simulink library "util_extra_lib"  (R2014b)
settings: Solver=ode45  StartTime=0.0  StopTime=10.0  RelTol=1e-3
values from neighbouring files (symbols this model uses):
  dt = 0.1    [quat_prop_test.m]
undefined symbols (not defined in the file or in its folder): duty_dt, min_dt, Newton, Raphson
undefined symbols (not defined in the file): asq_sequencer_rate, csc_gdn_dt, csu_rbd_orientation_prep_pitch_transfer_den, csu_rbd_orientation_prep_pitch_transfer_num
libraries: simulink x9, util_extra_lib x5, util_common_lib x1
settings Model: Creator=ianmga  LastModifiedBy=mstewart

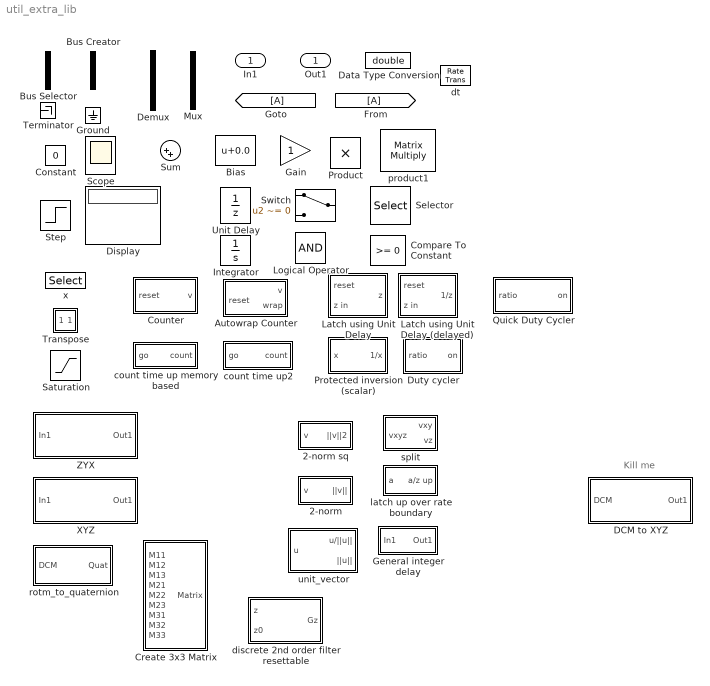
== system util_extra_lib ==
  note: Kill me
  In1 : Inport
  2-norm : Subsystem
  2-norm sq : Subsystem
  Autowrap Counter : Subsystem  mask{dt=dt, v0=int32( 0 ), dv=int32( 1 ), vlimit=int32( duty_dt / dt )}
      mask prompts: dt "Sample rate [s]"; v0 "Initial value"; dv "Increment"; vlimit "Wrap limit"
  Bias : Bias  Bias=0.0
  Bus Creator : BusCreator  Inputs=2
  Bus Selector : BusSelector  OutputSignals=signal1,signal2
  Compare To Constant : simulink/Logic and Bit Operations/Compare To Constant  relop=>=  const=0  OutDataTypeStr=uint8
  Constant : Constant  Value=0
  Counter : Subsystem  mask{dt=csc_gdn_dt, v0=0, dv=csc_gdn_dt}
      mask prompts: dt "Sample rate [s]"; v0 "Initial value"; dv "Increment"
  Create 3x3 Matrix : Subsystem  mask(Create 3x3 Matrix){}
      mask help:
      | Create a 3-by-3 matrix from nine input values. Each input corresponds to an element of the matrix.
      |
      | For example, the input labeled A21 is the entry in the second row and first column of the matrix.
      mask Help: eval('asbhelp(''create_threebythree_matrix'')');
      mask Display:
      | port_label('input',1,'A_{11}','texmode','on');
      | port_label('input',2,'A_{12}','texmode','on');
      | port_label('input',3,'A_{13}','texmode','on');
      | port_label('input',4,'A_{21}','texmode','on');
      | port_label('input',5,'A_{22}','texmode','on');
      | port_label('input',6,'A_{23}','texmode','on');
      | port_label('input',7,'A_{31}','texmode','on');
      | port_label('input',8,'A_{32}','texmode','on');
      | port_label('input',9,'A_{33}','texmode','on');
      | port_label('output',1,'A','texmode','on');
  DCM to XYZ : Subsystem  mask(DCM2Ang){}
      mask help:
      | Determine rotation vector from the 3-by-3 direction cosine matrix (DCM).
      |
      | The 'Default' limitations for the 'ZYX', 'ZXY', 'YXZ', 'YZX', 'XYZ', and 'XZY' implementations generate an R2 angle that lies between +/- 90 degrees, and R1 and R3 angles that lie between +/- 180 degrees.
      |
      | The 'Default' limitations for the 'ZYZ', 'ZXZ', 'YXY', 'YZY', 'XYX', and 'XZX' implementations generate an R2 angle that lies between 0 and 180 degrees, and R1 and R3 angles that lie between +/- 180 degrees.
      |
      | The 'ZeroR3' limitations for the 'ZYX', 'ZXY', 'YXZ', 'YZX', 'XYZ', and 'XZY' implementations generate an R2 angle that lies between +/- 90 degrees, and R1 and R3 angles that lie between +/- 180 degrees. However, when R2 is +/- 90 degrees, R3 is set to 0 degrees.
      |
      | The 'ZeroR3' limitations for the 'ZYZ', 'ZXZ', 'YXY', 'YZY', 'XYX', and 'XZX' implementations generate an R2 angle that lies between 0 and 180 degrees, and R1 and R3 angles that lie between +/- 180 degrees. However, when R2 is 0 or +/- 180 degrees, R3 is set to 0 degrees.
      mask Display:
      | port_label('input',1,'DCM^B_I','texmode','on')
      | port_label('output',1,'[R_X,R_Y,R_Z]','texmode','on')
  Data Type Conversion : DataTypeConversion  OutDataTypeStr=double
  Demux : Demux  Outputs=3
  Display : Display
  Duty cycler : Subsystem  mask{duty_dt=duty_dt, min_dt=min_dt, dt=dt}
      mask prompts: duty_dt "Duty cycle time [s]"; min_dt "Min duty cycle time [s]"; dt "Sample time [s]"
  Gain : Gain
  General integer delay : Subsystem  mask{delay_n=-1/.01, v0=0.0, dt=.01}
      mask prompts: delay_n "Delay samples"; v0 "Initial value"; dt "Sample time"
      mask Display:
      | port_label('input',1,'z');
      | port_label('output',1,'z^{-n}','texmode','on');
  Ground : Ground
  Integrator : Integrator
  Latch using Unit Delay : Subsystem  mask{z0=`, dt=dt}
      mask prompts: z0 "Initial value"; dt "Sample time"
  Latch using Unit Delay (delayed) : Subsystem  mask{z0=0, dt=dt}
      mask prompts: z0 "Initial value"; dt "Sample time"
  Logical Operator : Logic  AllPortsSameDT=off  OutDataTypeStr=boolean
  Mux : Mux  Inputs=3
  Product : Product  RndMeth=Zero
  Protected inversion (scalar) : Subsystem  mask{eps=1e-10}
  Quick Duty Cycler : Subsystem  mask{min_dt=0.1, dt=0.1}
      mask prompts: min_dt "Min duty cycle time [s]"; dt "Sample time [s]"
  Saturation : Saturate
  Scope : Scope  NumInputPorts=3
      settings: YMin=-5~-5~-5  YMax=5~5~5
  Selector : Selector  InputPortWidth=3  Indices=[1 3]
  Step : Step  SampleTime=0
  Sum : Sum  Inputs=|++
  Switch : Switch  Criteria=u2 ~= 0
  Terminator : Terminator
  Transpose : Subsystem  mask(Transpose){Hermitian=off, overflowFlag=off}
      mask prompts: overflowFlag "Saturate on integer overflow"
      mask help: Compute the matrix transpose. Vector input signals are treated as [Mx1] matrices. The output is always a matrix.
      mask init:
      | if(Hermitian==1)
      |     str = 'u^H';
      |     set_param([gcb '/Math Function'],'Operator','hermitian');
      |     if (overflowFlag==1)
      |         set_param([gcb '/Math Function'],'SaturateOnIntegerOverflow','on');
      |     else
      |         set_param([gcb '/Math Function'],'SaturateOnIntegerOverflow','off');
      |     end
      | else
      |     str = 'u^T';
      |     set_param([gcb '/Math Function'],'Operator','transpose');
      | end
      mask Help: eval('blocksethelp');
      mask Callback Hermitian:
      | if (strcmp(get_param(gcbh,'Hermitian'),'on'))
      | 	set_param(gcbh,'MaskVisibilities',{'on','on'});
      | else
      | 	set_param(gcbh,'MaskVisibilities',{'on','off'});
      | end
      mask Display: disp(str,'texmode','on')
  Unit Delay : UnitDelay  SampleTime=-1
  XYZ : Subsystem  mask(Ang2DCM){}
      mask help: Determine the 3-by-3 direction cosine matrix (DCM) from a given set of rotation angles.
      mask Display:
      | port_label('input',1,'[R_X,R_Y,R_Z]','texmode','on')
      | port_label('output',1,'DCM^B_I','texmode','on')
  ZYX : Subsystem  mask(Ang2DCM){}
      mask help: Determine the 3-by-3 direction cosine matrix (DCM) from a given set of rotation angles.
      mask Display:
      | port_label('input',1,'[R_Z,R_Y,R_X]','texmode','on')
      | port_label('output',1,'DCM^B_I','texmode','on')
  count time up memory based : Subsystem  mask{incr=int32( 1 ), v0=int32( 0 )}
      mask prompts: incr "Increment"; v0 "Initial value"
  count time up2 : Subsystem  mask{incr=asq_sequencer_rate, v0=0.0, dt=asq_sequencer_rate}
      mask prompts: incr "Increment"; v0 "Initial value"; dt "Sample time step"
  discrete 2nd order filter resettable : Subsystem  mask{num=csu_rbd_orientation_prep_pitch_transfer_num, den=csu_rbd_orientation_prep_pitch_transfer_den, dt=-1}
      mask prompts: num "Transfer fn numerator coefficients (bi)"; den "Transfer fn denominator coefficients (ai) (a1=1)"; dt "Sample rate (s)"
  dt : RateTransition  OutPortSampleTime=csc_gdn_dt
  latch up over rate boundary : Subsystem  mask{dt=.01}
      mask prompts: dt "Output sample time"
  product1 : Product  Multiplication=Matrix(*)
  rotm_to_quaternion : Subsystem  mask(DCM2Quaternion){}
      mask help: Determine the 4x1 quaternion orientation vector from a 3-by-3 direction cosine matrix (DCM). The input DCM transforms vectors from geodetic earth or north-east-down (NED) axes to body axes.
      mask Display:
      | port_label('output',1,'q^B_A','texmode','on')
      | port_label('input',1,'rotm^B_A','texmode','on')
  "split " : Subsystem
      mask Display:
      | port_label('input',1,'v_3','texmode','on')
      | port_label('output',1,'v_{xy}','texmode','on')
      | port_label('output',2,'v_z','texmode','on')
  unit_vector : Subsystem
      mask Display:
      | color('blue')
      | text(0.05,0.02,'NASA',...
      |  	'HorizontalAlignment','Left',...
      | 	'VerticalAlignment','bottom')
  x : Selector  InputPortWidth=3  Indices=[1]
  Out1 : Outport

== system util_extra_lib/2-norm ==
  v : Inport
  2-norm sq : util_extra_lib/2-norm sq
  Math Function : Math  Operator=sqrt  SaturateOnIntegerOverflow=on
  ||v|| : Outport
  wires:
  Math Function/1 -> ||v||/1
  v/1 -> 2-norm sq/1
  2-norm sq/1 -> Math Function/1

== system util_extra_lib/2-norm sq ==
  v : Inport
  Dot Product : DotProduct  InputSameDT=on  OutDataTypeStr=Inherit: Inherit via internal rule
  ||v||2 : Outport
  wires:
  Dot Product/1 -> ||v||2/1
  v/1 -> Dot Product/1, Dot Product/2

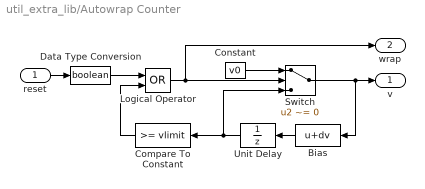
== system util_extra_lib/Autowrap Counter ==
  reset : Inport
  Bias : Bias  Bias=dv
  Compare To Constant : simulink/Logic and Bit Operations/Compare To Constant  relop=>=  const=vlimit  OutDataTypeStr=boolean
  Constant : Constant  Value=v0
  Data Type Conversion : DataTypeConversion  OutDataTypeStr=boolean
  Logical Operator : Logic  Operator=OR  AllPortsSameDT=off  OutDataTypeStr=boolean
  Switch : Switch  Criteria=u2 ~= 0  InputSameDT=on
  Unit Delay : UnitDelay  InitialCondition=vlimit  SampleTime=dt
  v : Outport
  wrap : Outport  Port=2
  wires:
  Data Type Conversion/1 -> Logical Operator/1
  Logical Operator/1 -> wrap/1, Switch/2
  reset/1 -> Data Type Conversion/1
  Compare To Constant/1 -> Logical Operator/2
  Constant/1 -> Switch/1
  Switch/1 -> Bias/1, v/1
  Bias/1 -> Unit Delay/1
  Unit Delay/1 -> Compare To Constant/1, Switch/3

== system util_extra_lib/Counter ==
  reset : Inport
  Bias : Bias  Bias=dv
  Constant : Constant  Value=v0  SampleTime=dt
  Switch : Switch  Criteria=u2 ~= 0  InputSameDT=on
  Unit Delay : UnitDelay  InitialCondition=v0  SampleTime=dt
  v : Outport
  wires:
  reset/1 -> Switch/2
  Unit Delay/1 -> Switch/3
  Bias/1 -> Unit Delay/1
  Switch/1 -> v/1, Bias/1
  Constant/1 -> Switch/1

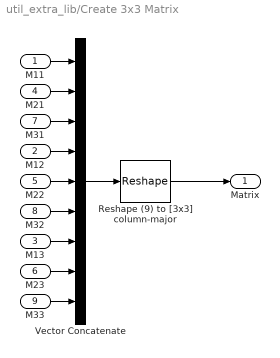
== system util_extra_lib/Create 3x3 Matrix ==
  M11 : Inport  PortDimensions=1
  M12 : Inport  Port=2  PortDimensions=1
  M13 : Inport  Port=3  PortDimensions=1
  M21 : Inport  Port=4  PortDimensions=1
  M22 : Inport  Port=5  PortDimensions=1
  M23 : Inport  Port=6  PortDimensions=1
  M31 : Inport  Port=7  PortDimensions=1
  M32 : Inport  Port=8  PortDimensions=1
  M33 : Inport  Port=9  PortDimensions=1
  Reshape (9) to [3x3] column-major : Reshape  OutputDimensionality=Customize  OutputDimensions=[3,3]
  Vector Concatenate : Concatenate  NumInputs=9
  Matrix : Outport  PortDimensions=[3 3]
  wires:
  M33/1 -> Vector Concatenate/9
  M23/1 -> Vector Concatenate/8
  M13/1 -> Vector Concatenate/7
  M32/1 -> Vector Concatenate/6
  Reshape (9) to [3x3] column-major/1 -> Matrix/1
  M22/1 -> Vector Concatenate/5
  M12/1 -> Vector Concatenate/4
  M31/1 -> Vector Concatenate/3
  M21/1 -> Vector Concatenate/2
  M11/1 -> Vector Concatenate/1
  Vector Concatenate/1 -> Reshape (9) to [3x3] column-major/1

== system util_extra_lib/DCM to XYZ ==
  DCM : Inport
  Abs : Abs
  AxisRotDefault : Subsystem
  AxisRotZeroR3 : Subsystem
  Get DCM Values : Subsystem
  Selector4 : Selector  InputPortWidth=7  Indices=3
  Switch : Switch  Threshold=1.0
  Out1 : Outport
  wires:
  Get DCM Values/1(Out1) -> AxisRotDefault/1(In1), AxisRotZeroR3/1(In1), Selector4/1
  AxisRotZeroR3/1(Out1) -> Switch/1
  AxisRotDefault/1(Out1) -> Switch/3
  Switch/1 -> Out1/1
  Abs/1 -> Switch/2
  Selector4/1 -> Abs/1  "r21"
  DCM/1 -> Get DCM Values/1(In1)

== system util_extra_lib/Duty cycler ==
  ratio : Inport
  Autowrap Counter : util_extra_lib/Autowrap Counter  SystemSampleTime=-1  dt=dt  v0=int32( 0 )  dv=int32( 1 )  vlimit=int32( duty_dt / dt )
  Constant2 : Constant  Value=false
  Gain : Gain  Gain=int32( duty_dt/min_dt )  OutDataTypeStr=int32
  Gain1 : Gain  Gain=int32( min_dt / dt )  OutDataTypeStr=int32
  Latch using Unit Delay : util_extra_lib/Latch using Unit Delay  SystemSampleTime=-1  z0=0  dt=dt
  Relational Operator : RelationalOperator  Operator=>  OutDataTypeStr=boolean
  on : Outport
  wires:
  Constant2/1 -> Autowrap Counter/1
  Gain/1 -> Gain1/1
  Relational Operator/1 -> on/1
  ratio/1 -> Latch using Unit Delay/2
  Latch using Unit Delay/1 -> Gain/1
  Autowrap Counter/1 -> Relational Operator/2
  Gain1/1 -> Relational Operator/1
  Autowrap Counter/2 -> Latch using Unit Delay/1

== system util_extra_lib/General integer delay ==
  In1 : Inport
  Constant : Constant  Value=delay_n
  Integer Delay1 : simulink/Discrete/Integer Delay  NumDelays=max( 1, delay_n )  vinit=v0  samptime=dt
  Switch1 : Switch  Criteria=u2 > Threshold
  Out1 : Outport
  wires:
  Switch1/1 -> Out1/1
  In1/1 -> Integer Delay1/1, Switch1/3
  Integer Delay1/1 -> Switch1/1
  Constant/1 -> Switch1/2

== system util_extra_lib/Latch using Unit Delay ==
  reset : Inport  SampleTime=dt
  z in : Inport  Port=2  SampleTime=dt
  Switch : Switch  Threshold=0.5  InputSameDT=on
  unit delay : UnitDelay  InitialCondition=z0  SampleTime=dt
  z : Outport
  wires:
  reset/1 -> Switch/2
  z in/1 -> Switch/1
  Switch/1 -> z/1, unit delay/1
  unit delay/1 -> Switch/3

== system util_extra_lib/Latch using Unit Delay (delayed) ==
  reset : Inport  SampleTime=dt
  z in : Inport  Port=2  SampleTime=dt
  Switch : Switch  Criteria=u2 ~= 0  Threshold=0.5
  unit delay : UnitDelay  InitialCondition=z0  SampleTime=dt
  1/z : Outport
  wires:
  Switch/1 -> unit delay/1
  unit delay/1 -> 1/z/1, Switch/3
  z in/1 -> Switch/1
  reset/1 -> Switch/2

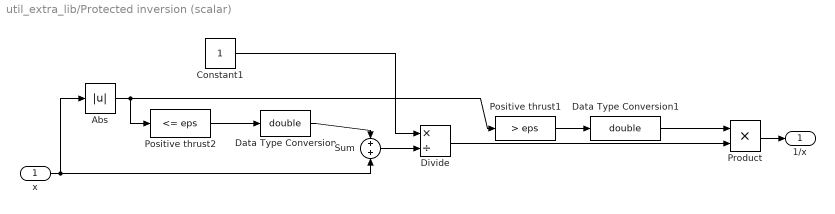
== system util_extra_lib/Protected inversion (scalar) ==
  x : Inport
  Abs : Abs
  Constant1 : Constant
  Data Type Conversion : DataTypeConversion  OutDataTypeStr=double
  Data Type Conversion1 : DataTypeConversion  OutDataTypeStr=double
  Divide : Product  Inputs=*/
  Positive thrust1 : simulink/Logic and Bit Operations/Compare To Constant  SystemSampleTime=-1  relop=>  const=eps  LogicOutDataTypeMode=uint8  ZeroCross=off
  Positive thrust2 : simulink/Logic and Bit Operations/Compare To Constant  SystemSampleTime=-1  relop=<=  const=eps  LogicOutDataTypeMode=uint8  ZeroCross=off
  Product : Product  RndMeth=Zero
  Sum : Sum  Inputs=+|+
  1/x : Outport
  wires:
  Positive thrust1/1 -> Data Type Conversion1/1
  Positive thrust2/1 -> Data Type Conversion/1
  Sum/1 -> Divide/2
  Constant1/1 -> Divide/1
  Divide/1 -> Product/2
  Data Type Conversion1/1 -> Product/1
  Product/1 -> 1/x/1
  x/1 -> Sum/2, Abs/1
  Abs/1 -> Positive thrust1/1, Positive thrust2/1
  Data Type Conversion/1 -> Sum/1

== system util_extra_lib/Quick Duty Cycler ==
  ratio : Inport
  Compare To Constant : simulink/Logic and Bit Operations/Compare To Constant  relop=<=  const=min_dt  OutDataTypeStr=boolean
  Compare To Constant1 : simulink/Logic and Bit Operations/Compare To Constant  relop=>  const=0  OutDataTypeStr=boolean
  Constant : Constant
  Discrete-Time Integrator : DiscreteIntegrator  ExternalReset=rising  SampleTime=dt
  Logical Operator : Logic  AllPortsSameDT=off  OutDataTypeStr=boolean
  Switch2 : Switch  Criteria=u2 ~= 0
  on : Outport
  wires:
  Logical Operator/1 -> Switch2/2
  Compare To Constant1/1 -> Logical Operator/2
  Compare To Constant/1 -> Logical Operator/1
  Constant/1 -> Switch2/1
  Discrete-Time Integrator/1 -> Compare To Constant/1, Compare To Constant1/1
  ratio/1 -> Discrete-Time Integrator/1, Switch2/3, Discrete-Time Integrator/2
  Switch2/1 -> on/1

== system util_extra_lib/Transpose ==
  In1 : Inport
  Math Function : Math  Operator=transpose  SaturateOnIntegerOverflow=on
  Out1 : Outport
  wires:
  Math Function/1 -> Out1/1
  In1/1 -> Math Function/1

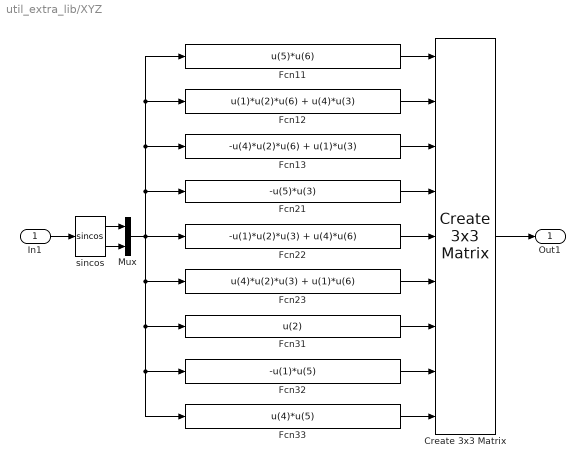
== system util_extra_lib/XYZ ==
  In1 : Inport  PortDimensions=3
  Create 3x3 Matrix : util_extra_lib/Create 3x3 Matrix  SystemSampleTime=-1
  Fcn11 : Fcn  Expr=u(5)*u(6)
  Fcn12 : Fcn  Expr=u(1)*u(2)*u(6) + u(4)*u(3)
  Fcn13 : Fcn  Expr=-u(4)*u(2)*u(6) + u(1)*u(3)
  Fcn21 : Fcn  Expr=-u(5)*u(3)
  Fcn22 : Fcn  Expr=-u(1)*u(2)*u(3) + u(4)*u(6)
  Fcn23 : Fcn  Expr=u(4)*u(2)*u(3) + u(1)*u(6)
  Fcn31 : Fcn  Expr=u(2)
  Fcn32 : Fcn  Expr=-u(1)*u(5)
  Fcn33 : Fcn  Expr=u(4)*u(5)
  Mux : Mux  Inputs=2
  sincos : Trigonometry  Operator=sincos
  Out1 : Outport  PortDimensions=[3,3]
  wires:
  In1/1 -> sincos/1
  Create 3x3 Matrix/1 -> Out1/1
  sincos/1 -> Mux/1
  sincos/2 -> Mux/2
  Mux/1 -> Fcn32/1, Fcn33/1, Fcn31/1, Fcn23/1, Fcn22/1, Fcn11/1, Fcn12/1, Fcn13/1, Fcn21/1
  Fcn11/1 -> Create 3x3 Matrix/1
  Fcn12/1 -> Create 3x3 Matrix/2
  Fcn13/1 -> Create 3x3 Matrix/3
  Fcn21/1 -> Create 3x3 Matrix/4
  Fcn31/1 -> Create 3x3 Matrix/7
  Fcn22/1 -> Create 3x3 Matrix/5
  Fcn23/1 -> Create 3x3 Matrix/6
  Fcn32/1 -> Create 3x3 Matrix/8
  Fcn33/1 -> Create 3x3 Matrix/9

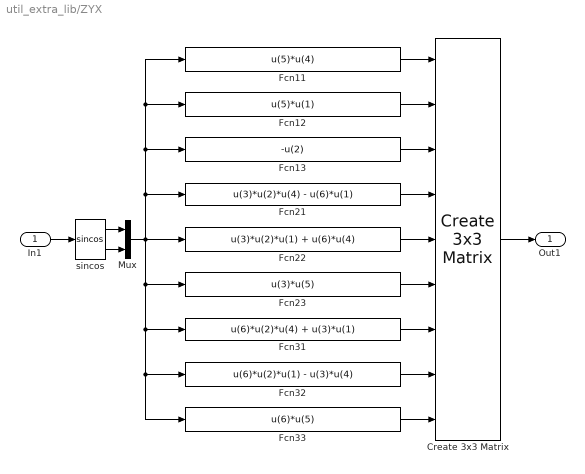
== system util_extra_lib/ZYX ==
  In1 : Inport  PortDimensions=3
  Create 3x3 Matrix : util_extra_lib/Create 3x3 Matrix  SystemSampleTime=-1
  Fcn11 : Fcn  Expr=u(5)*u(4)
  Fcn12 : Fcn  Expr=u(5)*u(1)
  Fcn13 : Fcn  Expr=-u(2)
  Fcn21 : Fcn  Expr=u(3)*u(2)*u(4) - u(6)*u(1)
  Fcn22 : Fcn  Expr=u(3)*u(2)*u(1) + u(6)*u(4)
  Fcn23 : Fcn  Expr=u(3)*u(5)
  Fcn31 : Fcn  Expr=u(6)*u(2)*u(4) + u(3)*u(1)
  Fcn32 : Fcn  Expr=u(6)*u(2)*u(1) - u(3)*u(4)
  Fcn33 : Fcn  Expr=u(6)*u(5)
  Mux : Mux  Inputs=2
  sincos : Trigonometry  Operator=sincos
  Out1 : Outport  PortDimensions=[3,3]
  wires:
  Fcn33/1 -> Create 3x3 Matrix/9
  Fcn32/1 -> Create 3x3 Matrix/8
  Fcn23/1 -> Create 3x3 Matrix/6
  Fcn22/1 -> Create 3x3 Matrix/5
  Fcn31/1 -> Create 3x3 Matrix/7
  Fcn21/1 -> Create 3x3 Matrix/4
  Fcn13/1 -> Create 3x3 Matrix/3
  Fcn12/1 -> Create 3x3 Matrix/2
  Fcn11/1 -> Create 3x3 Matrix/1
  Mux/1 -> Fcn21/1, Fcn13/1, Fcn12/1, Fcn11/1, Fcn22/1, Fcn23/1, Fcn31/1, Fcn33/1, Fcn32/1
  sincos/2 -> Mux/2
  sincos/1 -> Mux/1
  Create 3x3 Matrix/1 -> Out1/1
  In1/1 -> sincos/1

== system util_extra_lib/count time up memory based ==
  go : Inport
  Bias : Bias  Bias=incr
  Constant : Constant  Value=v0
  Memory : Memory  X0=v0  InheritSampleTime=on
  Switch : Switch  Criteria=u2 ~= 0  Threshold=0.5
  count : Outport
  wires:
  Constant/1 -> Switch/3
  Switch/1 -> Memory/1, count/1
  Bias/1 -> Switch/1
  go/1 -> Switch/2
  Memory/1 -> Bias/1

== system util_extra_lib/count time up2 ==
  go : Inport
  Bias : Bias  Bias=incr
  Constant : Constant  Value=v0  SampleTime=dt
  Switch : Switch  Criteria=u2 ~= 0  Threshold=0.5
  unit delay 1 : UnitDelay  InitialCondition=v0  SampleTime=dt
  count : Outport
  wires:
  go/1 -> Switch/2
  Switch/1 -> count/1, unit delay 1/1
  Constant/1 -> Switch/3
  unit delay 1/1 -> Bias/1
  Bias/1 -> Switch/1

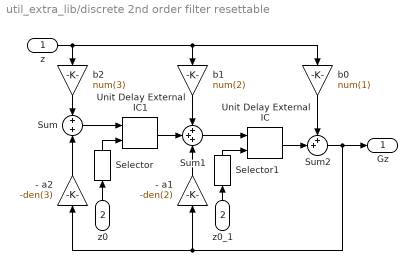
== system util_extra_lib/discrete 2nd order filter resettable ==
  z : Inport
  z0 : Inport  Port=2
  - a1 : Gain  Gain=-den(2)
  - a2 : Gain  Gain=-den(3)
  Selector : Selector  InputPortWidth=2  Indices=[2]
  Selector1 : Selector  InputPortWidth=2  Indices=[1]
  Sum : Sum  Inputs=+|+
  Sum1 : Sum  Inputs=+++
  Sum2 : Sum  Inputs=++|
  Unit Delay External IC : simulink/Additional Math & Discrete/Additional Discrete/Unit Delay External IC  SystemSampleTime=-1  tsamp=dt
  Unit Delay External IC1 : simulink/Additional Math & Discrete/Additional Discrete/Unit Delay External IC  SystemSampleTime=-1  tsamp=dt
  b0 : Gain  Gain=num(1)
  b1 : Gain  Gain=num(2)
  b2 : Gain  Gain=num(3)
  z0_1 : InportShadow  Port=2
  Gz : Outport
  wires:
  Sum2/1 -> - a2/1, - a1/1, Gz/1
  - a1/1 -> Sum1/3
  b0/1 -> Sum2/1
  Unit Delay External IC/1 -> Sum2/2
  b1/1 -> Sum1/1
  Sum1/1 -> Unit Delay External IC/1
  b2/1 -> Sum/1
  - a2/1 -> Sum/2
  Unit Delay External IC1/1 -> Sum1/2
  Sum/1 -> Unit Delay External IC1/1
  z/1 -> b0/1, b1/1, b2/1
  Selector1/1 -> Unit Delay External IC/2
  Selector/1 -> Unit Delay External IC1/2
  z0_1/1 -> Selector1/1
  z0/1 -> Selector/1

== system util_extra_lib/latch up over rate boundary ==
  a : Inport
  Logical Operator1 : Logic  Operator=OR  AllPortsSameDT=off  OutDataTypeStr=boolean
  Rate Transition1 : RateTransition  OutPortSampleTime=dt
  Unit Delay : UnitDelay  InitialCondition=dt  SampleTime=-1
  catcher : Subsystem  mask{z0=0, dt=-1}
      mask prompts: z0 "Initial value"; dt "Sample time"
  a/z up : Outport
  wires:
  Logical Operator1/1 -> catcher/1(reset)
  a/1 -> catcher/2(z in), Logical Operator1/2
  catcher/1(z) -> Rate Transition1/1
  Rate Transition1/1 -> a/z up/1, Unit Delay/1
  Unit Delay/1 -> Logical Operator1/1

== system util_extra_lib/rotm_to_quaternion ==
  DCM : Inport  PortDimensions=[3,3]
  If : If
  Merge : Merge
  Negative Trace : Subsystem  TreatAsAtomicUnit=on
  Positive Trace : Subsystem  TreatAsAtomicUnit=on
  "Reshape 3x3 -> 9" : Reshape  OutputDimensions=[9,1]
  trace(DCM) : Subsystem
  Quat : Outport  PortDimensions=4
  wires:
  Merge/1 -> Quat/1
  Positive Trace/1(qx qy qz qw) -> Merge/1
  trace(DCM)/1(trace(DCM)) -> Positive Trace/1(trace(DCM)), If/1
  "Reshape 3x3 -> 9"/1 -> trace(DCM)/1(DCM), Negative Trace/1(DCM), Positive Trace/2(DCM)
  DCM/1 -> "Reshape 3x3 -> 9"/1
  Negative Trace/1(qx qy qz qw) -> Merge/2
  If/1 -> Positive Trace/Action
  If/2 -> Negative Trace/Action

== system util_extra_lib/split  ==
  vxyz : Inport
  vxy cmd1 : Selector  InputPortWidth=3  Indices=[1 2]
  vz cmd1 : Selector  InputPortWidth=3  Indices=[3]
  vxy : Outport
  vz : Outport  Port=2
  wires:
  vz cmd1/1 -> vz/1
  vxy cmd1/1 -> vxy/1
  vxyz/1 -> vz cmd1/1, vxy cmd1/1

== system util_extra_lib/unit_vector ==
  u : Inport
  If : If  IfExpression=u1 ~= 0
  If Action Subsystem : Subsystem  TreatAsAtomicUnit=on
  Merge : Merge
  divide by zero detected : Subsystem  TreatAsAtomicUnit=on
  vector_magnitude : util_common_lib/vector_magnitude  SystemSampleTime=-1
  u/||u|| : Outport
  ||u|| : Outport  Port=2
  wires:
  Merge/1 -> u/||u||/1
  divide by zero detected/1(Out1) -> Merge/2
  If Action Subsystem/1(Out1) -> Merge/1
  If/2 -> divide by zero detected/Action
  If/1 -> If Action Subsystem/Action
  vector_magnitude/1 -> If Action Subsystem/2(In2), If/1, ||u||/1
  u/1 -> vector_magnitude/1, divide by zero detected/1(In1), If Action Subsystem/1(In1)

== system util_extra_lib/DCM to XYZ/AxisRotDefault ==
  In1 : Inport
  Fcn1 : Fcn  Expr=atan2(u[1],u[2])
  Fcn2 : Fcn  Expr=asin(u[3])
  Fcn3 : Fcn  Expr=atan2(u[4],u[5])
  Vector Concatenate : Concatenate  NumInputs=3
  Out1 : Outport
  wires:
  Vector Concatenate/1 -> Out1/1
  Fcn3/1 -> Vector Concatenate/3  "r3"
  Fcn2/1 -> Vector Concatenate/2  "r2"
  Fcn1/1 -> Vector Concatenate/1  "r1"
  In1/1 -> Fcn3/1, Fcn1/1, Fcn2/1

== system util_extra_lib/DCM to XYZ/AxisRotZeroR3 ==
  In1 : Inport
  Fcn1 : Fcn  Expr=atan2(u[6],u[7])
  Fcn2 : Fcn  Expr=asin(u[3])
  Fcn3 : Fcn  Expr=0
  Vector Concatenate : Concatenate  NumInputs=3
  Out1 : Outport
  wires:
  In1/1 -> Fcn2/1, Fcn1/1, Fcn3/1
  Fcn1/1 -> Vector Concatenate/1  "r1"
  Fcn2/1 -> Vector Concatenate/2  "r2"
  Fcn3/1 -> Vector Concatenate/3  "r3"
  Vector Concatenate/1 -> Out1/1

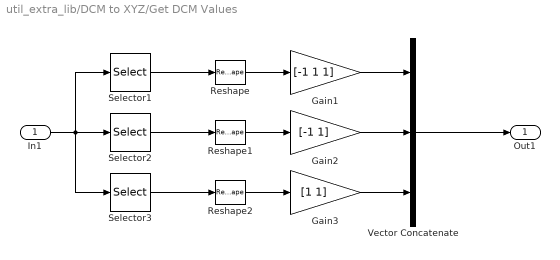
== system util_extra_lib/DCM to XYZ/Get DCM Values ==
  In1 : Inport
  Gain1 : Gain  Gain=[-1 1 1]
  Gain2 : Gain  Gain=[-1 1]
  Gain3 : Gain  Gain=[1 1]
  Reshape : Reshape
  Reshape1 : Reshape
  Reshape2 : Reshape
  Selector1 : Selector  NumberOfDimensions=2  InputPortWidth=3  IndexOptions=Index vector (dialog),Index vector (dialog)  Indices=3,[2 3 1]  OutputSizes=1,1
  Selector2 : Selector  NumberOfDimensions=2  InputPortWidth=3  IndexOptions=Index vector (dialog),Index vector (dialog)  Indices=[2 1],1  OutputSizes=1,1
  Selector3 : Selector  NumberOfDimensions=2  InputPortWidth=3  IndexOptions=Index vector (dialog),Index vector (dialog)  Indices=2,[3 2]  OutputSizes=1,1
  Vector Concatenate : Concatenate  NumInputs=3
  Out1 : Outport
  wires:
  Vector Concatenate/1 -> Out1/1
  Gain3/1 -> Vector Concatenate/3
  Gain2/1 -> Vector Concatenate/2
  Gain1/1 -> Vector Concatenate/1
  In1/1 -> Selector3/1, Selector2/1, Selector1/1
  Reshape2/1 -> Gain3/1
  Reshape1/1 -> Gain2/1
  Reshape/1 -> Gain1/1
  Selector1/1 -> Reshape/1
  Selector2/1 -> Reshape1/1
  Selector3/1 -> Reshape2/1

== system util_extra_lib/latch up over rate boundary/catcher ==
  reset : Inport  SampleTime=dt
  z in : Inport  Port=2  SampleTime=dt
  Switch : Switch  Threshold=0.5
  unit delay : UnitDelay  InitialCondition=z0  SampleTime=dt
  z : Outport
  wires:
  reset/1 -> Switch/2
  z in/1 -> Switch/1
  Switch/1 -> z/1, unit delay/1
  unit delay/1 -> Switch/3

== system util_extra_lib/rotm_to_quaternion/Negative Trace ==
  DCM : Inport
  Action Port : ActionPort
  Find Maximum Diagonal Value : If  NumInputs=3  IfExpression=((u2 > u1) & (u2 > u3))  ElseIfExpressions=u3 > u1
  Maximum Value at DCM(1,1) : Subsystem  TreatAsAtomicUnit=on
  Maximum Value at DCM(2,2) : Subsystem  TreatAsAtomicUnit=on
  Maximum Value at DCM(3,3) : Subsystem  TreatAsAtomicUnit=on
  Merge1 : Merge  Inputs=3
  diag(DCM) : Subsystem
  qx qy qz qw : Outport
  wires:
  Find Maximum Diagonal Value/2 -> Maximum Value at DCM(3,3)/Action
  Find Maximum Diagonal Value/1 -> Maximum Value at DCM(2,2)/Action
  Merge1/1 -> qx qy qz qw/1
  Maximum Value at DCM(1,1)/1(qx qy qz qw) -> Merge1/3
  Maximum Value at DCM(3,3)/1(qx qy qz qw) -> Merge1/2
  Maximum Value at DCM(2,2)/1(qx qy qz qw) -> Merge1/1
  Find Maximum Diagonal Value/3 -> Maximum Value at DCM(1,1)/Action
  DCM/1 -> diag(DCM)/1(DCM), Maximum Value at DCM(1,1)/1(DCM), Maximum Value at DCM(3,3)/1(DCM), Maximum Value at DCM(2,2)/1(DCM)
  diag(DCM)/1(u(1)) -> Find Maximum Diagonal Value/1
  diag(DCM)/2(u(5)) -> Find Maximum Diagonal Value/2
  diag(DCM)/3(u(9)) -> Find Maximum Diagonal Value/3

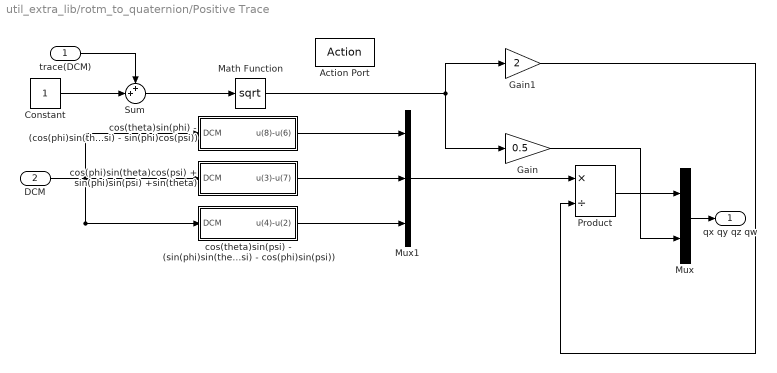
== system util_extra_lib/rotm_to_quaternion/Positive Trace ==
  trace(DCM) : Inport
  DCM : Inport  Port=2
  Action Port : ActionPort
  Constant : Constant  OutDataTypeStr=Inherit: Inherit via back propagation
  Gain : Gain  Gain=0.5  OutDataTypeStr=Inherit: Inherit via back propagation  SaturateOnIntegerOverflow=on  ParamDataTypeStr=Inherit: Same as input
  Gain1 : Gain  Gain=2  OutDataTypeStr=Inherit: Inherit via back propagation  SaturateOnIntegerOverflow=on  ParamDataTypeStr=Inherit: Same as input
  Math Function : Math  Operator=sqrt  SaturateOnIntegerOverflow=on
  Mux : Mux  Inputs=2
  Mux1 : Mux  Inputs=3
  Product : Product  Inputs=*/  SaturateOnIntegerOverflow=on  InputSameDT=on  OutDataTypeStr=Inherit: Same as first input
  Sum : Sum  Inputs=++|  SaturateOnIntegerOverflow=on  InputSameDT=on  OutDataTypeStr=Inherit: Same as first input
  cos(phi)sin(theta)cos(psi) + sin(phi)sin(psi) +sin(theta) : Subsystem
  cos(theta)sin(phi) - (cos(phi)sin(theta)sin(psi) - sin(phi)cos(psi)) : Subsystem
  cos(theta)sin(psi) - (sin(phi)sin(theta)cos(psi) - cos(phi)sin(psi)) : Subsystem
  qx qy qz qw : Outport
  wires:
  Gain/1 -> Mux/2
  Product/1 -> Mux/1
  trace(DCM)/1 -> Sum/1
  Constant/1 -> Sum/2
  Gain1/1 -> Product/2
  Mux1/1 -> Product/1
  DCM/1 -> cos(theta)sin(psi) - (sin(phi)sin(theta)cos(psi) - cos(phi)sin(psi))/1(DCM), cos(phi)sin(theta)cos(psi) + sin(phi)sin(psi) +sin(theta)/1(DCM), cos(theta)sin(phi) - (cos(phi)sin(theta)sin(psi) - sin(phi)cos(psi))/1(DCM)
  cos(theta)sin(phi) - (cos(phi)sin(theta)sin(psi) - sin(phi)cos(psi))/1(u(8)-u(6)) -> Mux1/1
  cos(phi)sin(theta)cos(psi) + sin(phi)sin(psi) +sin(theta)/1(u(3)-u(7)) -> Mux1/2
  cos(theta)sin(psi) - (sin(phi)sin(theta)cos(psi) - cos(phi)sin(psi))/1(u(4)-u(2)) -> Mux1/3
  Mux/1 -> qx qy qz qw/1
  Sum/1 -> Math Function/1
  Math Function/1 -> Gain/1, Gain1/1

== system util_extra_lib/rotm_to_quaternion/trace(DCM) ==
  DCM : Inport
  Add : Sum  Inputs=+
  Selector : Selector  InputPortWidth=9  Indices=[1 5 9]
  trace(DCM) : Outport
  wires:
  Selector/1 -> Add/1
  Add/1 -> trace(DCM)/1
  DCM/1 -> Selector/1

== system util_extra_lib/unit_vector/If Action Subsystem ==
  In1 : Inport
  In2 : Inport  Port=2
  Action Port : ActionPort
  Divide : Product  Inputs=*/
  Out1 : Outport
  wires:
  Divide/1 -> Out1/1
  In2/1 -> Divide/2
  In1/1 -> Divide/1

== system util_extra_lib/unit_vector/divide by zero detected ==
  In1 : Inport
  Action Port : ActionPort
  Out1 : Outport
  wires:
  In1/1 -> Out1/1

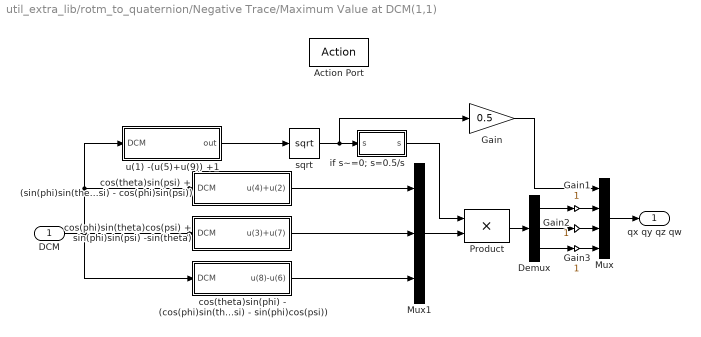
== system util_extra_lib/rotm_to_quaternion/Negative Trace/Maximum Value at DCM(1,1) ==
  DCM : Inport
  Action Port : ActionPort
  Demux : Demux  Outputs=3
  Gain : Gain  Gain=0.5  SaturateOnIntegerOverflow=on  OutDataTypeStr=Inherit: Same as input  ParamDataTypeStr=Inherit: Same as input
  Gain1 : Gain  SaturateOnIntegerOverflow=on  OutDataTypeStr=Inherit: Same as input  ParamDataTypeStr=Inherit: Same as input
  Gain2 : Gain  SaturateOnIntegerOverflow=on  OutDataTypeStr=Inherit: Same as input  ParamDataTypeStr=Inherit: Same as input
  Gain3 : Gain  SaturateOnIntegerOverflow=on  OutDataTypeStr=Inherit: Same as input  ParamDataTypeStr=Inherit: Same as input
  Mux : Mux
  Mux1 : Mux  Inputs=3
  Product : Product  SaturateOnIntegerOverflow=on  InputSameDT=on  OutDataTypeStr=Inherit: Same as first input
  cos(phi)sin(theta)cos(psi) + sin(phi)sin(psi) -sin(theta) : Subsystem
  cos(theta)sin(phi) - (cos(phi)sin(theta)sin(psi) - sin(phi)cos(psi)) : Subsystem
  cos(theta)sin(psi) + (sin(phi)sin(theta)cos(psi) - cos(phi)sin(psi)) : Subsystem
  if s~=0; s=0.5/s : Subsystem
  sqrt : Sqrt  AlgorithmType=Newton-Raphson  SaturateOnIntegerOverflow=on
  u(1) -(u(5)+u(9)) +1 : Subsystem
  qx qy qz qw : Outport
  wires:
  Gain3/1 -> Mux/4
  if s~=0; s=0.5/s/1("s ") -> Product/1
  Gain/1 -> Mux/1
  Product/1 -> Demux/1
  Gain2/1 -> Mux/3
  Gain1/1 -> Mux/2
  Demux/2 -> Gain2/1
  Demux/3 -> Gain3/1
  Demux/1 -> Gain1/1
  Mux1/1 -> Product/2
  sqrt/1 -> if s~=0; s=0.5/s/1(s), Gain/1
  u(1) -(u(5)+u(9)) +1/1(out) -> sqrt/1
  Mux/1 -> qx qy qz qw/1
  cos(theta)sin(phi) - (cos(phi)sin(theta)sin(psi) - sin(phi)cos(psi))/1(u(8)-u(6)) -> Mux1/3
  cos(phi)sin(theta)cos(psi) + sin(phi)sin(psi) -sin(theta)/1(u(3)+u(7)) -> Mux1/2
  cos(theta)sin(psi) + (sin(phi)sin(theta)cos(psi) - cos(phi)sin(psi))/1(u(4)+u(2)) -> Mux1/1
  DCM/1 -> u(1) -(u(5)+u(9)) +1/1(DCM), cos(theta)sin(psi) + (sin(phi)sin(theta)cos(psi) - cos(phi)sin(psi))/1(DCM), cos(theta)sin(phi) - (cos(phi)sin(theta)sin(psi) - sin(phi)cos(psi))/1(DCM), cos(phi)sin(theta)cos(psi) + sin(phi)sin(psi) -sin(theta)/1(DCM)

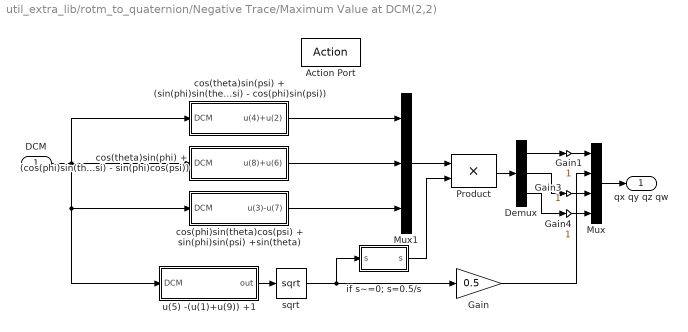
== system util_extra_lib/rotm_to_quaternion/Negative Trace/Maximum Value at DCM(2,2) ==
  DCM : Inport
  Action Port : ActionPort
  Demux : Demux  Outputs=3
  Gain : Gain  Gain=0.5  SaturateOnIntegerOverflow=on  OutDataTypeStr=Inherit: Same as input  ParamDataTypeStr=Inherit: Same as input
  Gain1 : Gain  SaturateOnIntegerOverflow=on  OutDataTypeStr=Inherit: Same as input  ParamDataTypeStr=Inherit: Same as input
  Gain3 : Gain  SaturateOnIntegerOverflow=on  OutDataTypeStr=Inherit: Same as input  ParamDataTypeStr=Inherit: Same as input
  Gain4 : Gain  SaturateOnIntegerOverflow=on  OutDataTypeStr=Inherit: Same as input  ParamDataTypeStr=Inherit: Same as input
  Mux : Mux
  Mux1 : Mux  Inputs=3
  Product : Product  SaturateOnIntegerOverflow=on  InputSameDT=on  OutDataTypeStr=Inherit: Same as first input
  cos(phi)sin(theta)cos(psi) + sin(phi)sin(psi) +sin(theta) : Subsystem
  cos(theta)sin(phi) + (cos(phi)sin(theta)sin(psi) - sin(phi)cos(psi)) : Subsystem
  cos(theta)sin(psi) + (sin(phi)sin(theta)cos(psi) - cos(phi)sin(psi)) : Subsystem
  if s~=0; s=0.5/s : Subsystem
  sqrt : Sqrt  AlgorithmType=Newton-Raphson  SaturateOnIntegerOverflow=on
  u(5) -(u(1)+u(9)) +1 : Subsystem
  qx qy qz qw : Outport
  wires:
  Gain4/1 -> Mux/4
  sqrt/1 -> Gain/1, if s~=0; s=0.5/s/1(s)
  if s~=0; s=0.5/s/1("s ") -> Product/2
  Gain3/1 -> Mux/3
  Gain1/1 -> Mux/1
  Demux/3 -> Gain4/1
  Demux/2 -> Gain3/1
  Demux/1 -> Gain1/1
  Product/1 -> Demux/1
  Gain/1 -> Mux/2
  u(5) -(u(1)+u(9)) +1/1(out) -> sqrt/1
  Mux/1 -> qx qy qz qw/1
  cos(phi)sin(theta)cos(psi) + sin(phi)sin(psi) +sin(theta)/1(u(3)-u(7)) -> Mux1/3
  cos(theta)sin(phi) + (cos(phi)sin(theta)sin(psi) - sin(phi)cos(psi))/1(u(8)+u(6)) -> Mux1/2
  cos(theta)sin(psi) + (sin(phi)sin(theta)cos(psi) - cos(phi)sin(psi))/1(u(4)+u(2)) -> Mux1/1
  DCM/1 -> u(5) -(u(1)+u(9)) +1/1(DCM), cos(phi)sin(theta)cos(psi) + sin(phi)sin(psi) +sin(theta)/1(DCM), cos(theta)sin(psi) + (sin(phi)sin(theta)cos(psi) - cos(phi)sin(psi))/1(DCM), cos(theta)sin(phi) + (cos(phi)sin(theta)sin(psi) - sin(phi)cos(psi))/1(DCM)
  Mux1/1 -> Product/1

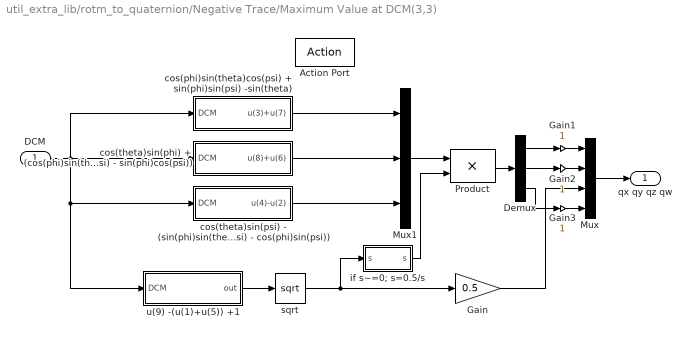
== system util_extra_lib/rotm_to_quaternion/Negative Trace/Maximum Value at DCM(3,3) ==
  DCM : Inport
  Action Port : ActionPort
  Demux : Demux  Outputs=3
  Gain : Gain  Gain=0.5  SaturateOnIntegerOverflow=on  OutDataTypeStr=Inherit: Same as input  ParamDataTypeStr=Inherit: Same as input
  Gain1 : Gain  SaturateOnIntegerOverflow=on  OutDataTypeStr=Inherit: Same as input  ParamDataTypeStr=Inherit: Same as input
  Gain2 : Gain  SaturateOnIntegerOverflow=on  OutDataTypeStr=Inherit: Same as input  ParamDataTypeStr=Inherit: Same as input
  Gain3 : Gain  SaturateOnIntegerOverflow=on  OutDataTypeStr=Inherit: Same as input  ParamDataTypeStr=Inherit: Same as input
  Mux : Mux
  Mux1 : Mux  Inputs=3
  Product : Product  SaturateOnIntegerOverflow=on  InputSameDT=on  OutDataTypeStr=Inherit: Same as first input
  cos(phi)sin(theta)cos(psi) + sin(phi)sin(psi) -sin(theta) : Subsystem
  cos(theta)sin(phi) + (cos(phi)sin(theta)sin(psi) - sin(phi)cos(psi)) : Subsystem
  cos(theta)sin(psi) - (sin(phi)sin(theta)cos(psi) - cos(phi)sin(psi)) : Subsystem
  if s~=0; s=0.5/s : Subsystem
  sqrt : Sqrt  AlgorithmType=Newton-Raphson  SaturateOnIntegerOverflow=on
  u(9) -(u(1)+u(5)) +1 : Subsystem
  qx qy qz qw : Outport
  wires:
  Gain3/1 -> Mux/4
  if s~=0; s=0.5/s/1("s ") -> Product/2
  Gain2/1 -> Mux/2
  Gain1/1 -> Mux/1
  Gain/1 -> Mux/3
  Demux/2 -> Gain2/1
  Demux/3 -> Gain3/1
  Demux/1 -> Gain1/1
  Product/1 -> Demux/1
  sqrt/1 -> if s~=0; s=0.5/s/1(s), Gain/1
  u(9) -(u(1)+u(5)) +1/1(out) -> sqrt/1
  Mux/1 -> qx qy qz qw/1
  cos(theta)sin(psi) - (sin(phi)sin(theta)cos(psi) - cos(phi)sin(psi))/1(u(4)-u(2)) -> Mux1/3
  cos(theta)sin(phi) + (cos(phi)sin(theta)sin(psi) - sin(phi)cos(psi))/1(u(8)+u(6)) -> Mux1/2
  cos(phi)sin(theta)cos(psi) + sin(phi)sin(psi) -sin(theta)/1(u(3)+u(7)) -> Mux1/1
  DCM/1 -> u(9) -(u(1)+u(5)) +1/1(DCM), cos(theta)sin(psi) - (sin(phi)sin(theta)cos(psi) - cos(phi)sin(psi))/1(DCM), cos(phi)sin(theta)cos(psi) + sin(phi)sin(psi) -sin(theta)/1(DCM), cos(theta)sin(phi) + (cos(phi)sin(theta)sin(psi) - sin(phi)cos(psi))/1(DCM)
  Mux1/1 -> Product/1

== system util_extra_lib/rotm_to_quaternion/Negative Trace/diag(DCM) ==
  DCM : Inport
  Demux : Demux  Outputs=3
  Selector : Selector  InputPortWidth=9  Indices=[1 5 9]
  u(1) : Outport
  u(5) : Outport  Port=2
  u(9) : Outport  Port=3
  wires:
  Selector/1 -> Demux/1
  Demux/3 -> u(9)/1
  Demux/2 -> u(5)/1
  Demux/1 -> u(1)/1
  DCM/1 -> Selector/1

== system util_extra_lib/rotm_to_quaternion/Positive Trace/cos(phi)sin(theta)cos(psi) + sin(phi)sin(psi) +sin(theta) ==
  DCM : Inport
  Add : Sum  Inputs=+-|
  Demux : Demux  Outputs=2
  Selector : Selector  InputPortWidth=9  Indices=[3 7]
  u(3)-u(7) : Outport
  wires:
  Demux/1 -> Add/1
  Demux/2 -> Add/2
  Selector/1 -> Demux/1
  Add/1 -> u(3)-u(7)/1
  DCM/1 -> Selector/1

== system util_extra_lib/rotm_to_quaternion/Positive Trace/cos(theta)sin(phi) - (cos(phi)sin(theta)sin(psi) - sin(phi)cos(psi)) ==
  DCM : Inport
  Add : Sum  Inputs=|-+
  Demux : Demux  Outputs=2
  Selector : Selector  InputPortWidth=9  Indices=[6 8]
  u(8)-u(6) : Outport
  wires:
  Selector/1 -> Demux/1
  Demux/2 -> Add/2
  Demux/1 -> Add/1
  DCM/1 -> Selector/1
  Add/1 -> u(8)-u(6)/1

== system util_extra_lib/rotm_to_quaternion/Positive Trace/cos(theta)sin(psi) - (sin(phi)sin(theta)cos(psi) - cos(phi)sin(psi)) ==
  DCM : Inport
  Add : Sum  Inputs=|-+
  Demux : Demux  Outputs=2
  Selector : Selector  InputPortWidth=9  Indices=[2 4]
  u(4)-u(2) : Outport
  wires:
  Demux/2 -> Add/2
  Demux/1 -> Add/1
  Selector/1 -> Demux/1
  DCM/1 -> Selector/1
  Add/1 -> u(4)-u(2)/1

== system util_extra_lib/rotm_to_quaternion/Negative Trace/Maximum Value at DCM(1,1)/cos(phi)sin(theta)cos(psi) + sin(phi)sin(psi) -sin(theta) ==
  DCM : Inport
  Add : Sum  Inputs=++|
  Demux : Demux  Outputs=2
  Selector : Selector  InputPortWidth=9  Indices=[3 7]
  u(3)+u(7) : Outport
  wires:
  Selector/1 -> Demux/1
  Demux/1 -> Add/1
  Demux/2 -> Add/2
  Add/1 -> u(3)+u(7)/1
  DCM/1 -> Selector/1

== system util_extra_lib/rotm_to_quaternion/Negative Trace/Maximum Value at DCM(1,1)/cos(theta)sin(phi) - (cos(phi)sin(theta)sin(psi) - sin(phi)cos(psi)) ==
  DCM : Inport
  Add : Sum  Inputs=|-+
  Demux : Demux  Outputs=2
  Selector : Selector  InputPortWidth=9  Indices=[6 8]
  u(8)-u(6) : Outport
  wires:
  Demux/2 -> Add/2
  Demux/1 -> Add/1
  Selector/1 -> Demux/1
  Add/1 -> u(8)-u(6)/1
  DCM/1 -> Selector/1

== system util_extra_lib/rotm_to_quaternion/Negative Trace/Maximum Value at DCM(1,1)/cos(theta)sin(psi) + (sin(phi)sin(theta)cos(psi) - cos(phi)sin(psi)) ==
  DCM : Inport
  Add : Sum  Inputs=|++
  Demux : Demux  Outputs=2
  Selector : Selector  InputPortWidth=9  Indices=[2 4]
  u(4)+u(2) : Outport
  wires:
  Demux/2 -> Add/2
  Demux/1 -> Add/1
  Selector/1 -> Demux/1
  DCM/1 -> Selector/1
  Add/1 -> u(4)+u(2)/1

== system util_extra_lib/rotm_to_quaternion/Negative Trace/Maximum Value at DCM(1,1)/if s~=0; s=0.5//s ==
  s : Inport
  Constant1 : Constant  Value=0.5  OutDataTypeStr=Inherit: Inherit via back propagation
  Constant2 : Constant  Value=[0 1]  OutDataTypeStr=Inherit: Inherit via back propagation
  Demux : Demux  Outputs=2
  Mux : Mux  Inputs=2
  Product : Product  Inputs=*/  RndMeth=Zero
  Switch : Switch  Criteria=u2 ~= 0  SaturateOnIntegerOverflow=on  InputSameDT=on
  "s " : Outport
  wires:
  Product/1 -> "s "/1
  Constant2/1 -> Switch/3
  Switch/1 -> Demux/1
  s/1 -> Mux/2, Switch/2
  Mux/1 -> Switch/1
  Constant1/1 -> Mux/1
  Demux/2 -> Product/2
  Demux/1 -> Product/1

== system util_extra_lib/rotm_to_quaternion/Negative Trace/Maximum Value at DCM(1,1)/u(1) -(u(5)+u(9)) +1 ==
  DCM : Inport
  Add : Sum  Inputs=+--+  InputSameDT=on
  Constant : Constant  OutDataTypeStr=Inherit: Inherit via back propagation
  Demux : Demux  Outputs=3
  Selector : Selector  InputPortWidth=9  Indices=[1 5 9]
  out : Outport
  wires:
  Demux/3 -> Add/3
  Demux/1 -> Add/1
  Demux/2 -> Add/2
  Selector/1 -> Demux/1
  Constant/1 -> Add/4
  DCM/1 -> Selector/1
  Add/1 -> out/1

== system util_extra_lib/rotm_to_quaternion/Negative Trace/Maximum Value at DCM(2,2)/cos(phi)sin(theta)cos(psi) + sin(phi)sin(psi) +sin(theta) ==
  DCM : Inport
  Add : Sum  Inputs=+-|
  Demux : Demux  Outputs=2
  Selector : Selector  InputPortWidth=9  Indices=[3 7]
  u(3)-u(7) : Outport
  wires:
  Selector/1 -> Demux/1
  Demux/1 -> Add/1
  DCM/1 -> Selector/1
  Demux/2 -> Add/2
  Add/1 -> u(3)-u(7)/1

== system util_extra_lib/rotm_to_quaternion/Negative Trace/Maximum Value at DCM(2,2)/cos(theta)sin(phi) + (cos(phi)sin(theta)sin(psi) - sin(phi)cos(psi)) ==
  DCM : Inport
  Add : Sum  Inputs=|++
  Demux : Demux  Outputs=2
  Selector : Selector  InputPortWidth=9  Indices=[6 8]
  u(8)+u(6) : Outport
  wires:
  Demux/2 -> Add/2
  Demux/1 -> Add/1
  Selector/1 -> Demux/1
  DCM/1 -> Selector/1
  Add/1 -> u(8)+u(6)/1

== system util_extra_lib/rotm_to_quaternion/Negative Trace/Maximum Value at DCM(2,2)/cos(theta)sin(psi) + (sin(phi)sin(theta)cos(psi) - cos(phi)sin(psi)) ==
  DCM : Inport
  Add : Sum  Inputs=|++
  Demux : Demux  Outputs=2
  Selector : Selector  InputPortWidth=9  Indices=[2 4]
  u(4)+u(2) : Outport
  wires:
  Demux/2 -> Add/2
  Demux/1 -> Add/1
  Selector/1 -> Demux/1
  Add/1 -> u(4)+u(2)/1
  DCM/1 -> Selector/1

== system util_extra_lib/rotm_to_quaternion/Negative Trace/Maximum Value at DCM(2,2)/if s~=0; s=0.5//s ==
  s : Inport
  Constant1 : Constant  Value=0.5  OutDataTypeStr=Inherit: Inherit via back propagation
  Constant2 : Constant  Value=[0 1]  OutDataTypeStr=Inherit: Inherit via back propagation
  Demux : Demux  Outputs=2
  Mux : Mux  Inputs=2
  Product : Product  Inputs=*/  RndMeth=Zero
  Switch : Switch  Criteria=u2 ~= 0  SaturateOnIntegerOverflow=on  InputSameDT=on
  "s " : Outport
  wires:
  Demux/1 -> Product/1
  Demux/2 -> Product/2
  Constant1/1 -> Mux/1
  Mux/1 -> Switch/1
  s/1 -> Switch/2, Mux/2
  Switch/1 -> Demux/1
  Constant2/1 -> Switch/3
  Product/1 -> "s "/1

== system util_extra_lib/rotm_to_quaternion/Negative Trace/Maximum Value at DCM(2,2)/u(5) -(u(1)+u(9)) +1 ==
  DCM : Inport
  Add : Sum  Inputs=-+-+  InputSameDT=on
  Constant : Constant  OutDataTypeStr=Inherit: Inherit via back propagation
  Demux : Demux  Outputs=3
  Selector : Selector  InputPortWidth=9  Indices=[1 5 9]
  out : Outport
  wires:
  Demux/3 -> Add/3
  Demux/1 -> Add/1
  Demux/2 -> Add/2
  Selector/1 -> Demux/1
  Add/1 -> out/1
  DCM/1 -> Selector/1
  Constant/1 -> Add/4

== system util_extra_lib/rotm_to_quaternion/Negative Trace/Maximum Value at DCM(3,3)/cos(phi)sin(theta)cos(psi) + sin(phi)sin(psi) -sin(theta) ==
  DCM : Inport
  Add : Sum  Inputs=++|
  Demux : Demux  Outputs=2
  Selector : Selector  InputPortWidth=9  Indices=[3 7]
  u(3)+u(7) : Outport
  wires:
  Selector/1 -> Demux/1
  Demux/1 -> Add/1
  Demux/2 -> Add/2
  DCM/1 -> Selector/1
  Add/1 -> u(3)+u(7)/1

== system util_extra_lib/rotm_to_quaternion/Negative Trace/Maximum Value at DCM(3,3)/cos(theta)sin(phi) + (cos(phi)sin(theta)sin(psi) - sin(phi)cos(psi)) ==
  DCM : Inport
  Add : Sum  Inputs=|++
  Demux : Demux  Outputs=2
  Selector : Selector  InputPortWidth=9  Indices=[6 8]
  u(8)+u(6) : Outport
  wires:
  Demux/2 -> Add/2
  Demux/1 -> Add/1
  Selector/1 -> Demux/1
  Add/1 -> u(8)+u(6)/1
  DCM/1 -> Selector/1

== system util_extra_lib/rotm_to_quaternion/Negative Trace/Maximum Value at DCM(3,3)/cos(theta)sin(psi) - (sin(phi)sin(theta)cos(psi) - cos(phi)sin(psi)) ==
  DCM : Inport
  Add : Sum  Inputs=|-+
  Demux : Demux  Outputs=2
  Selector : Selector  InputPortWidth=9  Indices=[2 4]
  u(4)-u(2) : Outport
  wires:
  Demux/2 -> Add/2
  Demux/1 -> Add/1
  Selector/1 -> Demux/1
  Add/1 -> u(4)-u(2)/1
  DCM/1 -> Selector/1

== system util_extra_lib/rotm_to_quaternion/Negative Trace/Maximum Value at DCM(3,3)/if s~=0; s=0.5//s ==
  s : Inport
  Constant1 : Constant  Value=0.5  OutDataTypeStr=Inherit: Inherit via back propagation
  Constant2 : Constant  Value=[0 1]  OutDataTypeStr=Inherit: Inherit via back propagation
  Demux : Demux  Outputs=2
  Mux : Mux  Inputs=2
  Product : Product  Inputs=*/  RndMeth=Zero
  Switch : Switch  Criteria=u2 ~= 0  SaturateOnIntegerOverflow=on  InputSameDT=on
  "s " : Outport
  wires:
  Product/1 -> "s "/1
  Constant2/1 -> Switch/3
  Switch/1 -> Demux/1
  s/1 -> Mux/2, Switch/2
  Mux/1 -> Switch/1
  Constant1/1 -> Mux/1
  Demux/2 -> Product/2
  Demux/1 -> Product/1

== system util_extra_lib/rotm_to_quaternion/Negative Trace/Maximum Value at DCM(3,3)/u(9) -(u(1)+u(5)) +1 ==
  DCM : Inport
  Add : Sum  Inputs=--++  InputSameDT=on
  Constant : Constant  OutDataTypeStr=Inherit: Inherit via back propagation
  Demux : Demux  Outputs=3
  Selector : Selector  InputPortWidth=9  Indices=[1 5 9]
  out : Outport
  wires:
  Demux/3 -> Add/3
  Demux/1 -> Add/1
  Demux/2 -> Add/2
  Selector/1 -> Demux/1
  Add/1 -> out/1
  DCM/1 -> Selector/1
  Constant/1 -> Add/4
